simulink model "oscdrag"  (Simulink 3.00)
settings: Solver=ode45  StartTime=0.0  StopTime=40  RelTol=1e-3
values from neighbouring files (symbols this model uses):
  kappa = rho*S*Cd/2    (= 0.007618)    [cannonballpar.m]    (also in pendragpar.m = 0.0003809)
  m = 1    [cannonballpar.m]    (also in pendcartpar.m; pendragpar.m = 0.01)
  W = 2    [pend4par.m]
  w = 1    [pendragpar.m]

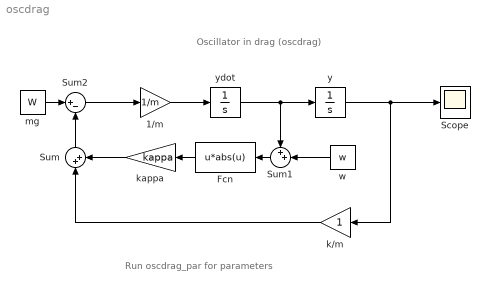
== system oscdrag ==
  note: Oscillator in drag (oscdrag)
  note: Run oscdrag_par for parameters
  1/m : Gain  Gain=1/m  SaturateOnIntegerOverflow=on
  Fcn : Fcn  Orientation=left  Expr=u*abs(u)
  Scope : Scope
      settings: TimeRange=auto  YMin=-5  YMax=5  SaveToWorkspace=off  SaveName=ScopeData
  Sum : Sum  Orientation=up  Inputs=|++  SaturateOnIntegerOverflow=on
  Sum1 : Sum  Orientation=left  Inputs=++|  SaturateOnIntegerOverflow=on
  Sum2 : Sum  Inputs=|+-  SaturateOnIntegerOverflow=on
  k/m : Gain  Orientation=left  Gain=1  SaturateOnIntegerOverflow=on
  kappa : Gain  Orientation=left  Gain=kappa  SaturateOnIntegerOverflow=on
  mg : Constant  Value=W
  w : Constant  Orientation=left  Value=w
  y : Integrator  ExternalReset=none  InitialConditionSource=internal  InitialCondition=0  LimitOutput=off  UpperSaturationLimit=inf  LowerSaturationLimit=-inf  ShowSaturationPort=off  ShowStatePort=off  AbsoluteTolerance=auto
  ydot : Integrator  ExternalReset=none  InitialConditionSource=internal  InitialCondition=0  LimitOutput=off  UpperSaturationLimit=inf  LowerSaturationLimit=-inf  ShowSaturationPort=off  ShowStatePort=off  AbsoluteTolerance=auto
  wires:
  y/1 -> k/m/1, Scope/1
  ydot/1 -> y/1, Sum1/1
  Sum1/1 -> Fcn/1
  w/1 -> Sum1/2
  1/m/1 -> ydot/1
  Fcn/1 -> kappa/1
  k/m/1 -> Sum/1
  Sum2/1 -> 1/m/1
  mg/1 -> Sum2/1
  kappa/1 -> Sum/2
  Sum/1 -> Sum2/2
